simulink model "main"  (R2022a)
settings: Solver=VariableStepAuto  StartTime=0.0  StopTime=10.0  RelTol=1e-3
settings Model: Creator=li_fe  LastModifiedBy=li_fe

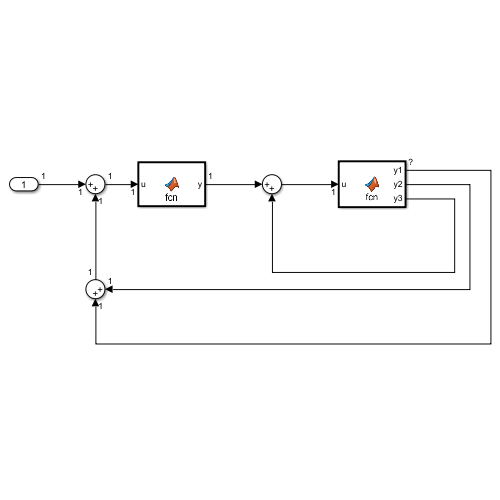
[thumbnail: Simulink's stored preview of the top-level diagram]
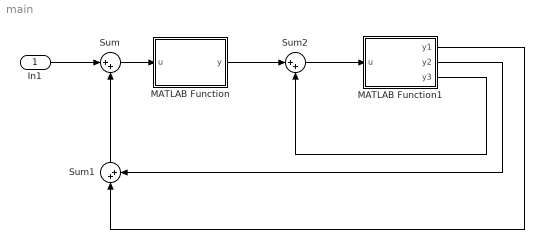
== system main ==
  In1 : Inport
  MATLAB Function : MATLAB Function  TreatAsAtomicUnit=on
  MATLAB Function1 : MATLAB Function  TreatAsAtomicUnit=on
  Sum : Sum  Inputs=|++
  Sum1 : Sum  Inputs=|++
  Sum2 : Sum  Inputs=|++
  wires:
  In1/1 -> Sum/1
  Sum/1 -> MATLAB Function/1(u)
  MATLAB Function1/1(y1) -> Sum1/1
  MATLAB Function1/2(y2) -> Sum1/2
  Sum1/1 -> Sum/2
  MATLAB Function/1(y) -> Sum2/1
  Sum2/1 -> MATLAB Function1/1(u)
  MATLAB Function1/3(y3) -> Sum2/2

== matlab function main/MATLAB Function ==
  data: u input; y output
function y = fcn(u)

y = [1,2,3];

== matlab function main/MATLAB Function1 ==
  data: y1 output; y2 output; y3 output; u input
function [y1, y2, y3]= fcn(u)
y1 = u(1);
y2 = u(2);
y3 = u(2);
